simulink model "SixDOF_Test"  (R2022a)
settings: Solver=VariableStepAuto  StartTime=0.0  StopTime=50  RelTol=1e-3
libraries: shared6dof x1
settings Model: Creator=ndelurgio  LastModifiedBy=ndelurgio

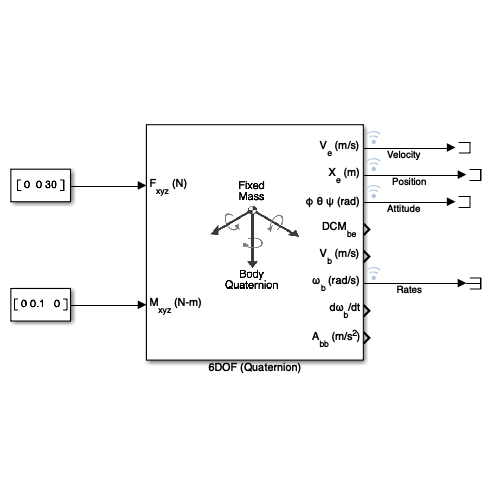
[thumbnail: Simulink's stored preview of the top-level diagram]
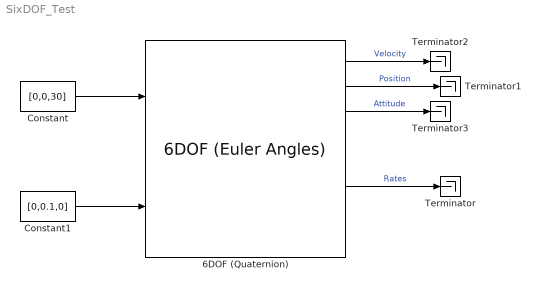
== system SixDOF_Test ==
  6DOF (Quaternion) : shared6dof/6DOF (Euler Angles)  units=Metric (MKS)  mtype=Fixed  rep=Quaternion  xme_0=[0 0 0]  Vm_0=[0 0 0]  eul_0=[0 0 0]  pm_0=[0 0 0]  mass_0=200  mass_e=0.5  mass_f=2.0  inertia=[100 10 0; 10 100 0; 0 0 200]  inertia_e=eye(3)  inertia_f=2*eye(3)  k_quat=1.0  vre_flag=on  abi_flag=off  aMode=0  xme_statename=''  Vm_statename=''  eul_statename=''  quat_statename=''  pm_statename=''  mass_statename=''
      settings: SourceProductBaseCode=AE,PW,DR,MT,VE
  Constant : Constant  Value=[0,0,30]
  Constant1 : Constant  Value=[0,0.1,0]
  Terminator{,1..3} (4 alike) : Terminator
  wires:
  Constant/1 -> 6DOF (Quaternion)/1
  Constant1/1 -> 6DOF (Quaternion)/2
  6DOF (Quaternion)/6 -> Terminator/1  "Rates"
  6DOF (Quaternion)/2 -> Terminator1/1  "Position"
  6DOF (Quaternion)/1 -> Terminator2/1  "Velocity"
  6DOF (Quaternion)/3 -> Terminator3/1  "Attitude"
